simulink model "simulator"  (Simulink 8.0)
settings: Solver=ode1  SolverMode=SingleTasking  StartTime=0.0  StopTime=0.5  FixedStep=0.001  RelTol=1e-3
values from neighbouring files (symbols this model uses):
  Beq = 0.0015    [Sve_ikad.m]    (also in matlab.mat)
  den_k = [1 100*a]    [Sve_ikad.m]
  Eff_G = 0.9    [Sve_ikad.m]    (also in matlab.mat)
  Eff_M = 0.69    [Sve_ikad.m]    (also in matlab.mat)
  Jeq = 9.785e-5    (= 9.785e-05)    [Sve_ikad.m]    (also in matlab.mat)
  Ke = 0.0076776    [Sve_ikad.m]    (also in matlab.mat)
  Kg = 14    [Sve_ikad.m]    (also in matlab.mat)
  Km = 0.007683    [Sve_ikad.m]    (also in matlab.mat)
  Kp = 41.55    [Sve_ikad.m]    (also in matlab.mat = 41.6)
  num_k = [1*a 100]    [Sve_ikad.m]
  Ra = 2.6    [Sve_ikad.m]    (also in matlab.mat)
settings Model: Creator=Labos  LastModifiedBy=Niko
settings DataIOCC: SignalLoggingSaveFormat=ModelDataLogs
settings DebuggingCC: FcnCallInpInsideContextMsg=UseLocalSettings  StrictBusMsg=Warning
settings GRTTargetCC: CombineOutputUpdateFcns=off  GRTInterface=on

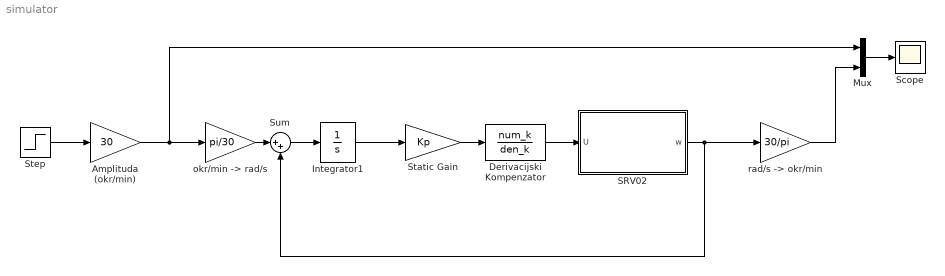
== system simulator ==
  Amplituda (okr/min) : Gain  Gain=30
  Derivacijski Kompenzator : TransferFcn  Numerator=num_k  Denominator=den_k
  Integrator1 : Integrator
  Mux : Mux  Inputs=2
  "SRV02 " : Subsystem
  Scope : Scope
      settings: TimeRange=5  YMin=0  YMax=30  SaveName=Response  SampleInput=on
  Static Gain : Gain  Gain=Kp
  Step : Step  Time=0.1  SampleTime=0.001
  Sum : Sum  Inputs=|++
  "okr/min -> rad/s" : Gain  Gain=pi/30
  "rad/s -> okr/min" : Gain  Gain=30/pi
  wires:
  "okr/min -> rad/s"/1 -> Sum/1
  Static Gain/1 -> Derivacijski Kompenzator/1
  "rad/s -> okr/min"/1 -> Mux/2
  Mux/1 -> Scope/1
  Step/1 -> Amplituda (okr/min)/1
  Amplituda (okr/min)/1 -> Mux/1, "okr/min -> rad/s"/1
  Sum/1 -> Integrator1/1
  Integrator1/1 -> Static Gain/1
  Derivacijski Kompenzator/1 -> "SRV02 "/1(U)
  "SRV02 "/1(w) -> Sum/2, "rad/s -> okr/min"/1

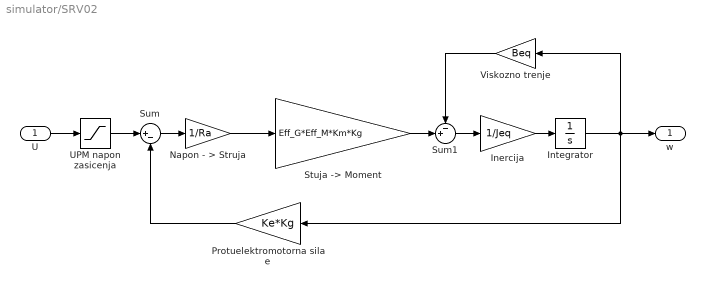
== system simulator/SRV02  ==
  U : Inport
  Inercija : Gain  Gain=1/Jeq
  Integrator : Integrator
  Napon - > Struja : Gain  Gain=1/Ra
  Protuelektromotorna sila e : Gain  Gain=Ke*Kg
  "Stuja -> Moment" : Gain  Gain=Eff_G*Eff_M*Km*Kg
  Sum : Sum  Inputs=|+-
  Sum1 : Sum  Inputs=-+|
  UPM napon zasicenja : Saturate  UpperLimit=6  LowerLimit=-6
  Viskozno trenje : Gain  Gain=Beq
  w : Outport
  wires:
  Sum1/1 -> Inercija/1
  "Stuja -> Moment"/1 -> Sum1/2
  Inercija/1 -> Integrator/1
  UPM napon zasicenja/1 -> Sum/1
  Napon - > Struja/1 -> "Stuja -> Moment"/1
  U/1 -> UPM napon zasicenja/1
  Sum/1 -> Napon - > Struja/1
  Viskozno trenje/1 -> Sum1/1
  Protuelektromotorna sila e/1 -> Sum/2
  Integrator/1 -> w/1, Protuelektromotorna sila e/1, Viskozno trenje/1
